simulink model "Common_Cathode_Configuration_of_Diode_Using_Simulink"  (R2021b)
settings: Solver=VariableStepAuto  StartTime=0.0  StopTime=10.0  RelTol=1e-3
undefined symbols (not defined in the file): Ts
libraries: spsControlledVoltageSourceLib x3, spsDiodeLib x3, spsMultimeterLib x1, spsSeriesRLCBranchLib x1, spspowerguiLib x1
settings Model: Creator=Vansh  LastModifiedBy=Vansh
settings DebuggingCC: UnconnectedInputMsg=none  UnconnectedOutputMsg=none  UnconnectedLineMsg=none

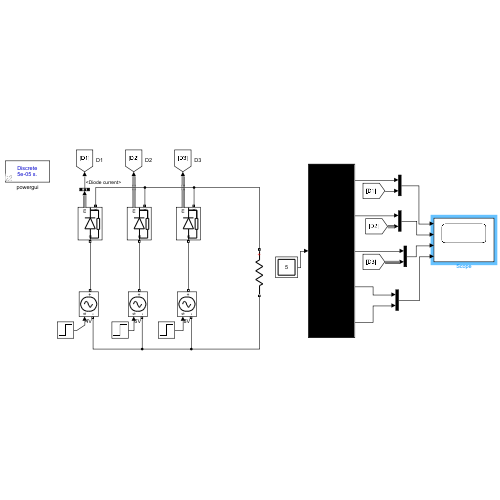
[thumbnail: Simulink's stored preview of the top-level diagram]
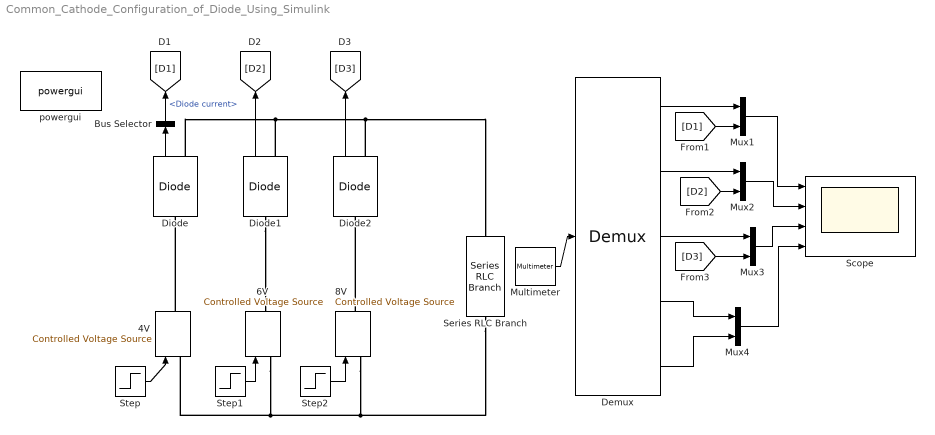
== system Common_Cathode_Configuration_of_Diode_Using_Simulink ==
  4V : spsControlledVoltageSourceLib/Controlled Voltage Source  Initialize=on  Source_Type=DC  Amplitude=10  Phase=0  Frequency=0  Measurements=Voltage
  6V : spsControlledVoltageSourceLib/Controlled Voltage Source  Initialize=on  Source_Type=DC  Amplitude=10  Phase=0  Frequency=0  Measurements=Voltage
  8V : spsControlledVoltageSourceLib/Controlled Voltage Source  Initialize=on  Source_Type=DC  Amplitude=10  Phase=0  Frequency=0  Measurements=Voltage
  Bus Selector : BusSelector  OutputSignals=Diode current
  Demux : Demux  Outputs=5
  Diode : spsDiodeLib/Diode  Ron=0.001  Lon=0  Vf=2  IC=0  UseSnubber=0  Rs=500  Cs=250e-9  Measurements=on
  Diode1 : spsDiodeLib/Diode  Ron=0.001  Lon=0  Vf=2  IC=0  UseSnubber=0  Rs=500  Cs=250e-9  Measurements=on
  Diode2 : spsDiodeLib/Diode  Ron=0.001  Lon=0  Vf=2  IC=0  UseSnubber=0  Rs=500  Cs=250e-9  Measurements=on
  Multimeter : spsMultimeterLib/Multimeter  PhasorSimulation=off  OutputType=Complex  sel=[2 3 4 1 5]  L=5  Gain=[1 1 1 1 1]  yselected={'Usrc: 4V','Usrc: 6V','Usrc: 8V','Ub: Series RLC Branch','Ib: Series RLC Branch'};  PSBOutputType=1  PSBequivalent=0  AxesSetting=[0,0.1,-100,100]  Display=0  SavedBlockNames=-11
  Mux{1..4} (4 alike) : Mux  Inputs=2
  Scope : Scope  NumInputPorts=4
  Series RLC Branch : spsSeriesRLCBranchLib/Series RLC Branch  LConnTagsString=__new0  RConnTagsString=__new0  BranchType=R  Resistance=2  Inductance=1e-3  SetiL0=off  InitialCurrent=0  Capacitance=1e-6  Setx0=off  InitialVoltage=0  Measurements=Branch voltage and current
  Step : Step  After=4  SampleTime=Ts
  Step1 : Step  Time=2  After=6  SampleTime=Ts
  Step2 : Step  Time=3  After=8  SampleTime=Ts
  powergui : spspowerguiLib/powergui  Priority=1  SimulationMode=Discrete  SampleTime=50e-6  frequency=60  Iterations=50  frequencyindice=0  Pbase=100e6  ErrMax=1e-4  UnitsV=kV  UnitsW=MW  buscounter=0  FunctionMessages=off  echomessages=off  EnableUseOfTLC=off  CurrentSourceSwitches=off  DisableSnubberDevices=off  DisableRonSwitches=off  DisableVfSwitches=off  DisplayEquations=off  AutomaticDiscreteSolvers=off  SolverType=Tustin/Backward Euler (TBE)  Interpol=off  ExternalGateDelay=off  methode=off  Ts=100  x0status=blocks  SPID=on  SwTol=0  HookPort=off  NonlinearTolerance=1e-4  nMaxIteration=100  ContinueOnMaxIteration=off  RestoreLinks=warning  ResistiveCurrentMeasurement=off  Frange=[0:2:500]  Ylog=off  Xlog=on  ShowGrid=off  save=off  variable=ZData  structure=0  ZoomFFT=off  StartTime=0.0  cycles=1  DisplayStyle=1  fundamental=60  FreqAxis=off  MaxFrequency=1000  frequencyindicesteady=1  RmsSteady=1  display=off
  wires:
  Step2/1 -> 8V/1
  Step1/1 -> 6V/1
  Diode/1 -> Bus Selector/1
  Step/1 -> 4V/1
  Bus Selector/1 -> [D1]  "<Diode current>"
  Diode2/1 -> [D3]
  Diode1/1 -> [D2]
  Multimeter/1 -> Demux/1
  Demux/1 -> Mux1/1
  [D1] -> Mux1/2
  [D2] -> Mux2/2
  Demux/2 -> Mux2/1
  Demux/3 -> Mux3/1
  [D3] -> Mux3/2
  Demux/4 -> Mux4/1
  Demux/5 -> Mux4/2
  Mux4/1 -> Scope/4
  Mux3/1 -> Scope/3
  Mux2/1 -> Scope/2
  Mux1/1 -> Scope/1
  connections:
  Series RLC Branch/RConn1 -- 8V/LConn1 -- 6V/LConn1 -- 4V/LConn1
  Diode/RConn1 -- Diode1/RConn1 -- Diode2/RConn1 -- Series RLC Branch/LConn1
  Diode1/LConn1 -- 6V/RConn1
  8V/RConn1 -- Diode2/LConn1
  4V/RConn1 -- Diode/LConn1
